simulink model "untitled"  (Simulink 7.3)
settings: Solver=ode45  StartTime=0.0  StopTime=10.0  RelTol=1e-3
settings Model: Creator=root  LastModifiedBy=root

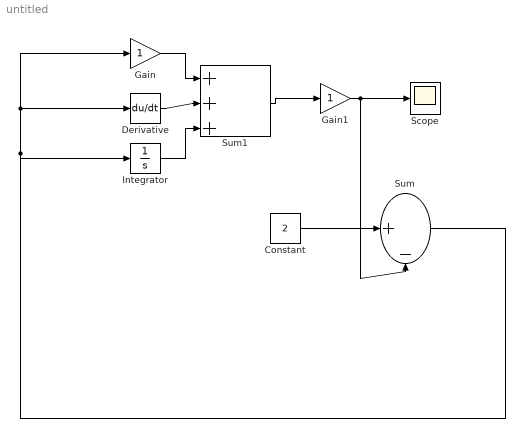
== system untitled ==
  Constant : Constant  Value=2  OutDataType=fixdt(1, 16)  OutScaling=2^0
  Derivative : Derivative
  Gain : Gain  ParameterDataType=fixdt(1, 16)  ParameterScaling=2^0  OutDataType=fixdt(1, 16)  OutScaling=2^0
  Gain1 : Gain  ParameterDataType=fixdt(1, 16)  ParameterScaling=2^0  OutDataType=fixdt(1, 16)  OutScaling=2^0
  Integrator : Integrator
  Scope : Scope
  Sum : Sum  Inputs=|+-  OutDataType=fixdt(1, 16)  OutScaling=2^0
  Sum1 : Sum  Inputs=|+++  OutDataType=fixdt(1, 16)  OutScaling=2^0
  wires:
  Gain/1 -> Sum1/1
  Derivative/1 -> Sum1/2
  Integrator/1 -> Sum1/3
  Sum1/1 -> Gain1/1
  Sum/1 -> Gain/1, Derivative/1, Integrator/1
  Constant/1 -> Sum/1
  Gain1/1 -> Scope/1, Sum/2
